simulink model "mains"  (R2021a)
settings: Solver=VariableStepAuto  StartTime=0.0  StopTime=100  RelTol=1e-4
values from neighbouring files (symbols this model uses):
  a = 1    [final_fusion.m]    (also in four_compass.m)
  b = 2*eta/w    (= 0.0512623349994)    [final_fusion.m]    (also in four_compass.m)
  c = 1/w^2    (= 0.153787004998)    [final_fusion.m]    (also in four_compass.m)
  d = k    (= 1)    [final_fusion.m]    (also in four_compass.m)
settings Model: Creator=zd012  LastModifiedBy=zd012

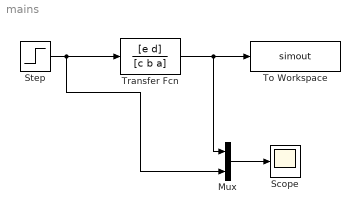
== system mains ==
  Mux : Mux  Inputs=2
  Scope : Scope
  Step : Step  Time=0  After=10  SampleTime=0
  To Workspace : ToWorkspace  VariableName=simout  SaveFormat=Timeseries  SampleTime=-1
  Transfer Fcn : TransferFcn  Numerator=[e d]  Denominator=[c b a]
  wires:
  Step/1 -> Mux/2, Transfer Fcn/1
  Transfer Fcn/1 -> Mux/1, To Workspace/1
  Mux/1 -> Scope/1
